simulink library "BatteryLib"  (R2020a)
settings: Solver=ode45  StartTime=0.0  StopTime=10.0  RelTol=1e-3  EnableMultiTasking=on
undefined symbols (not defined in the file): Battery, Env, magnitude
libraries: fl_lib x10, nesl_utility x5
settings Model: Creator=tbria  LastModifiedBy=Harjot
settings DataIOCC: LimitDataPoints=on  SaveFormat=Array
settings OptimizationCC: LifeSpan=inf
settings DebuggingCC: SFUnexpectedBacktrackingDiag=warning  SFNoUnconditionalDefaultTransitionDiag=warning  SFExecutionAtInitializationDiag=none  ArithmeticOperatorsInVariantConditions=warning
settings HardwareCC: ProdBitPerPointer=32  ProdBitPerSizeT=32  ProdBitPerPtrDiffT=32  ProdLargestAtomicFloat=None  ProdIntDivRoundTo=Undefined  ProdEndianess=Unspecified  ProdWordSize=32  ProdHWDeviceType=32-bit Generic
settings ModelReferenceCC: PropagateSignalLabelsOutOfModel=off
settings SFSimCC: SimUseLocalCustomCode=off  CustomCodeUndefinedFunction=UseInterfaceOnly
settings RTWCC: RTWUseLocalCustomCode=off
settings CodeAppCC: StateflowObjectComments=on
settings GRTTargetCC: TargetLangStandard=C89/C90 (ANSI)
settings ConfigComp: CovMetricSettings=dw  CovHtmlReporting=on  CovSaveCumulativeToWorkspaceVar=on  CovSaveSingleToWorkspaceVar=on  CovExternalEMLEnable=off

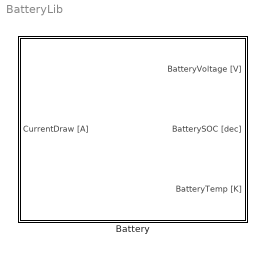
== system BatteryLib ==
  Battery : Subsystem

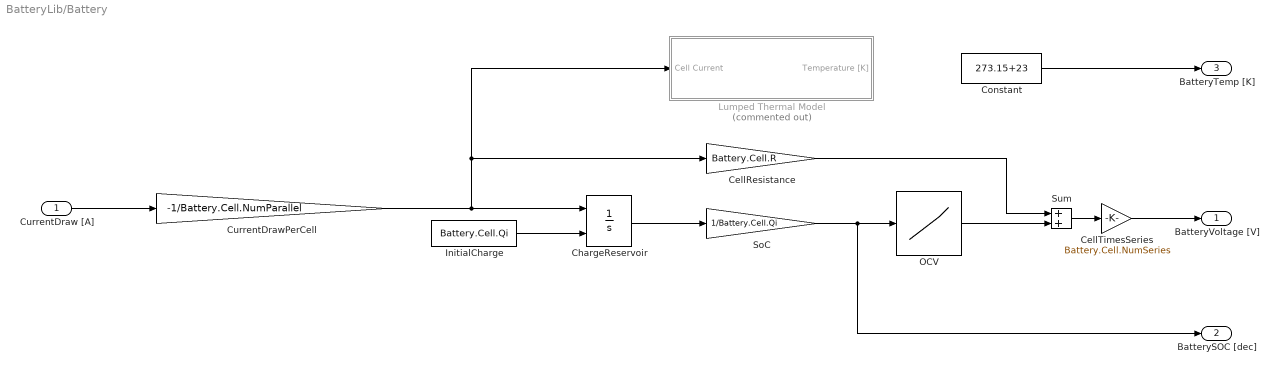
== system BatteryLib/Battery ==
  CurrentDraw [A] : Inport
  CellResistance : Gain  Gain=Battery.Cell.R
  CellTimesSeries : Gain  Gain=Battery.Cell.NumSeries
  ChargeReservoir : Integrator  InitialConditionSource=external
  Constant : Constant  Value=273.15+23
  CurrentDrawPerCell : Gain  Gain=-1/Battery.Cell.NumParallel
  InitialCharge : Constant  Value=Battery.Cell.Qi
  Lumped Thermal Model : Subsystem  Commented=on
  OCV : Lookup_n-D  NumberOfTableDimensions=1  BreakpointsForDimension1=Battery.Cell.VoltOC.SoC  Table=Battery.Cell.VoltOC.Voltage  InternalRulePriority=Speed  RndMeth=Simplest  InputSameDT=on
  SoC : Gain  Gain=1/Battery.Cell.Qi
  Sum : Sum
  BatteryVoltage [V] : Outport  VectorParamsAs1DForOutWhenUnconnected=off
  BatterySOC [dec] : Outport  Port=2  VectorParamsAs1DForOutWhenUnconnected=off
  BatteryTemp [K] : Outport  Port=3  VectorParamsAs1DForOutWhenUnconnected=off
  wires:
  Constant/1 -> BatteryTemp [K]/1
  CurrentDraw [A]/1 -> CurrentDrawPerCell/1
  InitialCharge/1 -> ChargeReservoir/2
  ChargeReservoir/1 -> SoC/1
  SoC/1 -> OCV/1, BatterySOC [dec]/1
  CellTimesSeries/1 -> BatteryVoltage [V]/1
  CellResistance/1 -> Sum/1
  OCV/1 -> Sum/2
  Sum/1 -> CellTimesSeries/1
  CurrentDrawPerCell/1 -> Lumped Thermal Model/1(Cell Current), CellResistance/1, ChargeReservoir/1

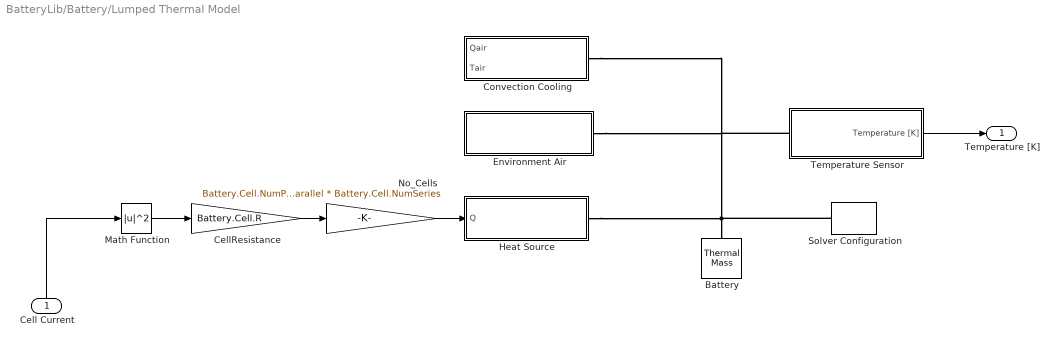
== system BatteryLib/Battery/Lumped Thermal Model ==
  Cell Current : Inport
  Battery : fl_lib/Thermal/Thermal Elements/Thermal Mass  mass=Battery.Cell.m*Battery.Cell.NumParallel * Battery.Cell.NumSeries kg  sp_heat=Battery.Cell.c J/kg/K  T_specify=off  T_priority=High  T=300 K  T_nominal_specify=off  T_nominal_unit=K  T_nominal_value=1  Q_specify=off  Q_priority=High  Q=0 J/s  Q_nominal_specify=off  Q_nominal_unit=W  Q_nominal_value=1
  CellResistance : Gain  Gain=Battery.Cell.R
  Convection Cooling : Subsystem
  Environment Air : Subsystem
  Heat Source : Subsystem
  Math Function : Math  Operator=magnitude^2  SignedPower=on  SaturateOnIntegerOverflow=on
  No_Cells : Gain  Gain=Battery.Cell.NumParallel * Battery.Cell.NumSeries
  Solver Configuration : nesl_utility/Solver Configuration  PhysicalDomain=network_engine_domain  SubClassName=solver  LeftPortType=input  RightPortType=generic  Tones=[]  Harmonics=[]  SimulateNoise=off  Profile=off  UseLocalSampling=off  EnableSwitchedLinearOptims=on  FrequencyDomain=off  UseCCode=off  RelTol=0.001  AbsTol=1e-06  MinStep=1e-09  ToWorkspace=off  RevertToSquareIcSolve=off  NumHomotopyIterations=100  PhasorMode=off  PhasorModeNumHarmonics=1  DoDC=off  ResidualTolerance=1e-09  UseLocalSolver=off  LocalSolverChoice=NE_BACKWARD_EULER_ADVANCER  LocalSolverSampleTime=0.001  DoFixedCost=off  MaxNonlinIter=3  MaxModeIter=2  LinearAlgebra=Sparse  EquationFormulation=NE_TIME_EF  DelaysMemoryBudget=1024  AutomaticFiltering=on  FilteringTimeConstant=0.001  PartitionStorageMethod=AS_NEEDED  PartitionMemoryBudget=1024  PartitionMethod=FAST
  Temperature Sensor : Subsystem
  Temperature [K] : Outport  VectorParamsAs1DForOutWhenUnconnected=off
  wires:
  Math Function/1 -> CellResistance/1
  CellResistance/1 -> No_Cells/1
  No_Cells/1 -> Heat Source/1(Q)
  Temperature Sensor/1(Temperature [K]) -> Temperature [K]/1
  Cell Current/1 -> Math Function/1
  connections:
  Heat Source/RConn1 -- Environment Air/RConn1 -- Temperature Sensor/LConn1 -- Convection Cooling/RConn1 -- Solver Configuration/RConn1 -- Battery/LConn1

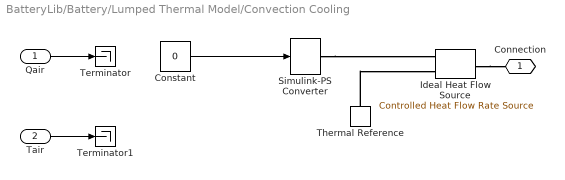
== system BatteryLib/Battery/Lumped Thermal Model/Convection Cooling ==
  Qair : Inport
  Tair : Inport  Port=2
  Constant : Constant  Value=0
  Ideal Heat Flow Source : fl_lib/Thermal/Thermal Sources/Controlled Heat Flow Rate Source
  Simulink-PS Converter : nesl_utility/Simulink-PS Converter  PhysicalDomain=network_engine_domain  SubClassName=ps_input  LeftPortType=input  RightPortType=output  PseudoPeriodic=off  Frequencies=[]  NoiseDistribution=none  NoiseParameters=[]  Unit=1  AffineConversion=off  FilteringAndDerivatives=zero  SimscapeFilterOrder=1  InputFilterTimeConstant=0.001  UdotUserProvided=1
  Terminator : Terminator
  Terminator1 : Terminator
  Thermal Reference : fl_lib/Thermal/Thermal Elements/Thermal Reference
  Connection : PMIOPort  Side=Right
  wires:
  Tair/1 -> Terminator1/1
  Qair/1 -> Terminator/1
  Constant/1 -> Simulink-PS Converter/1
  connections:
  Simulink-PS Converter/RConn1 -- Ideal Heat Flow Source/RConn1
  Thermal Reference/LConn1 -- Ideal Heat Flow Source/RConn2
  Ideal Heat Flow Source/LConn1 -- Connection/RConn1

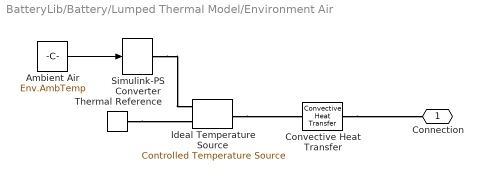
== system BatteryLib/Battery/Lumped Thermal Model/Environment Air ==
  Ambient Air : Constant  Value=Env.AmbTemp
  Convective Heat Transfer : fl_lib/Thermal/Thermal Elements/Convective Heat Transfer  area=Battery.SA m^2  heat_tr_coeff=Env.NaturalConvection.K W/(m^2 * K)  T_specify=off  T_priority=High  T=0 K  T_nominal_specify=off  T_nominal_unit=K  T_nominal_value=1  Q_specify=off  Q_priority=High  Q=0 J/s  Q_nominal_specify=off  Q_nominal_unit=W  Q_nominal_value=1
  Ideal Temperature Source : fl_lib/Thermal/Thermal Sources/Controlled Temperature Source
  Simulink-PS Converter : nesl_utility/Simulink-PS Converter  PhysicalDomain=network_engine_domain  SubClassName=ps_input  LeftPortType=input  RightPortType=output  PseudoPeriodic=off  Frequencies=[]  NoiseDistribution=none  NoiseParameters=[]  Unit=1  AffineConversion=off  FilteringAndDerivatives=zero  SimscapeFilterOrder=1  InputFilterTimeConstant=0.001  UdotUserProvided=1
  Thermal Reference : fl_lib/Thermal/Thermal Elements/Thermal Reference
  Connection : PMIOPort  Side=Right
  wires:
  Ambient Air/1 -> Simulink-PS Converter/1
  connections:
  Ideal Temperature Source/LConn1 -- Convective Heat Transfer/LConn1
  Simulink-PS Converter/RConn1 -- Ideal Temperature Source/RConn1
  Thermal Reference/LConn1 -- Ideal Temperature Source/RConn2
  Convective Heat Transfer/RConn1 -- Connection/RConn1

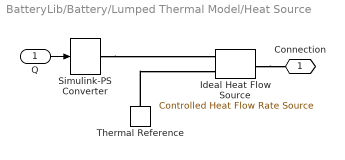
== system BatteryLib/Battery/Lumped Thermal Model/Heat Source ==
  Q : Inport
  Ideal Heat Flow Source : fl_lib/Thermal/Thermal Sources/Controlled Heat Flow Rate Source
  Simulink-PS Converter : nesl_utility/Simulink-PS Converter  PhysicalDomain=network_engine_domain  SubClassName=ps_input  LeftPortType=input  RightPortType=output  PseudoPeriodic=off  Frequencies=[]  NoiseDistribution=none  NoiseParameters=[]  Unit=1  AffineConversion=off  FilteringAndDerivatives=zero  SimscapeFilterOrder=1  InputFilterTimeConstant=0.001  UdotUserProvided=1
  Thermal Reference : fl_lib/Thermal/Thermal Elements/Thermal Reference
  Connection : PMIOPort  Side=Right
  wires:
  Q/1 -> Simulink-PS Converter/1
  connections:
  Simulink-PS Converter/RConn1 -- Ideal Heat Flow Source/RConn1
  Thermal Reference/LConn1 -- Ideal Heat Flow Source/RConn2
  Ideal Heat Flow Source/LConn1 -- Connection/RConn1

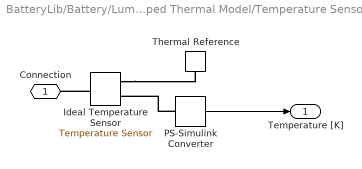
== system BatteryLib/Battery/Lumped Thermal Model/Temperature Sensor ==
  Ideal Temperature Sensor : fl_lib/Thermal/Thermal Sensors/Temperature Sensor
  PS-Simulink Converter : nesl_utility/PS-Simulink Converter  PhysicalDomain=network_engine_domain  SubClassName=ps_output  LeftPortType=input  RightPortType=output  PseudoPeriodic=off  Frequencies=[]  Unit=1  AffineConversion=off
  Thermal Reference : fl_lib/Thermal/Thermal Elements/Thermal Reference
  Connection : PMIOPort  Side=Left
  Temperature [K] : Outport  VectorParamsAs1DForOutWhenUnconnected=off
  wires:
  PS-Simulink Converter/1 -> Temperature [K]/1
  connections:
  Ideal Temperature Sensor/LConn1 -- Connection/RConn1
  PS-Simulink Converter/LConn1 -- Ideal Temperature Sensor/RConn2
  Ideal Temperature Sensor/RConn1 -- Thermal Reference/LConn1
